simulink model "exp3_5_STATE_SPACE_LQR_FREQ"  (R2020b)
settings: Solver=ode3  StartTime=0.0  StopTime=10  FixedStep=0.001  RelTol=1e-3
undefined symbols (not defined in the file): Aq, Bq, denH_w, DiscIntNeverNeededParam, enable_integral_action, K_ih, K_ss, National_Instruments, Nu, numH_w, Nx, PCI, sens, step_height, step_start_time, Ts
libraries: sldrtlib x3, simulink x3
settings Model: SimulationMode=external  ExtModeTrigDuration=150000  Creator=controlsystemsuser  LastModifiedBy=grandinmat
settings DataIOCC: ReturnWorkspaceOutputs=off
settings RTWCC: Description=Simulink Desktop Real-Time  SystemTargetFile=sldrt.tlc  TemplateMakefile=sldrt.tmf  RTWCompilerOptimization=on
settings CodeAppCC: MaxIdLength=95
settings SimulinkDesktopRealTimeCC: TargetPreCompLibLocation=C:\Program Files\MATLAB\R2020b\toolbox\sldrt\lib\win64

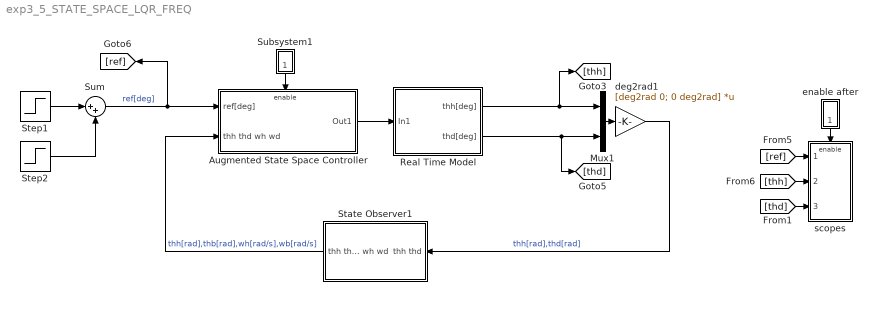
== system exp3_5_STATE_SPACE_LQR_FREQ ==
  Augmented State Space Controller : Subsystem
  Mux1 : Mux  Inputs=2
  Real Time Model : Subsystem
  State Observer1 : Subsystem
  Step1 : Step  Time=step_start_time  After=step_height  SampleTime=0
  Step2 : Step  Time=step_start_time+5  After=-step_height  SampleTime=0
  Subsystem1 : Subsystem
  Sum : Sum  Inputs=|++
  deg2rad1 : Gain  Gain=[deg2rad 0; 0 deg2rad]  Multiplication=Matrix(K*u) (u vector)
  enable after : Subsystem
  scopes : Subsystem
  wires:
  Step2/1 -> Sum/2
  Sum/1 -> Augmented State Space Controller/1(ref[deg]), [ref]  "ref[deg]"
  Step1/1 -> Sum/1
  State Observer1/1(thh thd wh wd) -> Augmented State Space Controller/2(thh thd wh wd)  "thh[rad],thb[rad],wh[rad/s],wb[rad/s]"
  Augmented State Space Controller/1(Out1) -> Real Time Model/1(In1)
  Mux1/1 -> deg2rad1/1
  deg2rad1/1 -> State Observer1/1(thh thd)  "thh[rad],thd[rad]"
  Subsystem1/1(0.8) -> Augmented State Space Controller/Enable
  Real Time Model/2(thd[deg]) -> [thd], Mux1/2
  Real Time Model/1(thh[deg]) -> [thh], Mux1/1
  [thh] -> scopes/2(thh[deg])
  [ref] -> scopes/1(ref[deg])
  [thd] -> scopes/3(thd[deg])
  enable after/1(1.0 s) -> scopes/Enable

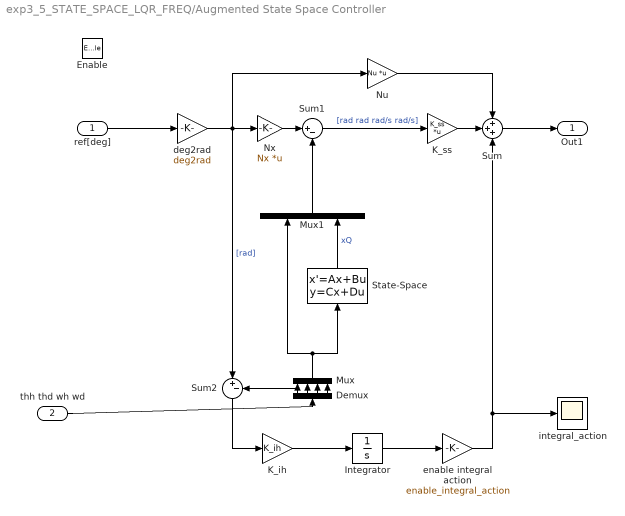
== system exp3_5_STATE_SPACE_LQR_FREQ/Augmented State Space Controller ==
  ref[deg] : Inport
  thh thd wh wd : Inport  Port=2
  Enable : EnablePort
  Demux : Demux
  Integrator : Integrator
  K_ih : Gain  Gain=K_ih
  K_ss : Gain  Gain=K_ss  Multiplication=Matrix(K*u) (u vector)
  Mux : Mux
  Mux1 : Mux  Inputs=2
  Nu : Gain  Gain=Nu  Multiplication=Matrix(K*u) (u vector)
  Nx : Gain  Gain=Nx  Multiplication=Matrix(K*u) (u vector)
  State-Space : StateSpace  A=Aq  B=Bq  C=eye(2,2)  D=zeros(2,4)  InitialCondition=0
  Sum : Sum  Inputs=+++
  Sum1 : Sum  Inputs=|+-
  Sum2 : Sum  Inputs=|+-
  deg2rad : Gain  Gain=deg2rad
  enable integral action : Gain  Gain=enable_integral_action
  integral_action : Scope
  Out1 : Outport
  wires:
  deg2rad/1 -> Nx/1, Nu/1, Sum2/1  "[rad]"
  K_ss/1 -> Sum/2
  Nx/1 -> Sum1/1
  ref[deg]/1 -> deg2rad/1
  Nu/1 -> Sum/1
  Sum/1 -> Out1/1
  Sum1/1 -> K_ss/1  "[rad rad rad/s rad/s]"
  Demux/1 -> Mux/1, Sum2/2
  Demux/2 -> Mux/2
  Demux/3 -> Mux/3
  Demux/4 -> Mux/4
  thh thd wh wd/1 -> Demux/1
  Sum2/1 -> K_ih/1
  enable integral action/1 -> Sum/3, integral_action/1
  Mux/1 -> State-Space/1, Mux1/1
  State-Space/1 -> Mux1/2  "xQ"
  Mux1/1 -> Sum1/2
  K_ih/1 -> Integrator/1
  Integrator/1 -> enable integral action/1

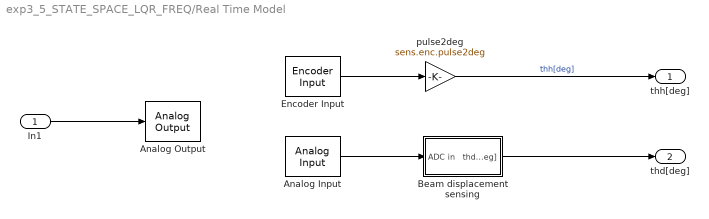
== system exp3_5_STATE_SPACE_LQR_FREQ/Real Time Model ==
  In1 : Inport
  Analog Input : sldrtlib/Analog Input  SampleTime=0.001  MaxMissedTicks=10  ShowMissedTicks=off  YieldWhenWaiting=off  DrvName=National_Instruments/PCI-6221  DrvAddress=4294967295  DrvOptions=[0 0 0 2 0]  Channels=[3,4]  RangeMode=1  VoltRange=2  DataType=1
      settings: AttributesFormatString=National Instruments\nPCI-6221 [auto]
  Analog Output : sldrtlib/Analog Output  SampleTime=0.001  MaxMissedTicks=10  ShowMissedTicks=off  YieldWhenWaiting=off  DrvName=National_Instruments/PCI-6221  DrvAddress=4294967295  DrvOptions=[0 0 0 2 0]  Channels=1  RangeMode=1  VoltRange=1  InitialValue=0  FinalValue=0
      settings: AttributesFormatString=National Instruments\nPCI-6221 [auto]
  Beam displacement sensing : Subsystem
  Encoder Input : sldrtlib/Encoder Input  SampleTime=0.001  MaxMissedTicks=10  ShowMissedTicks=off  YieldWhenWaiting=off  DrvName=National_Instruments/PCI-6221  DrvAddress=4294967295  DrvOptions=[0 0 0 2 0]  Channels=1  QuadMode=3  IndexPulse=1  InputFilter=Inf  DataType=1
      settings: AttributesFormatString=National Instruments\nPCI-6221 [auto]
  pulse2deg : Gain  Gain=sens.enc.pulse2deg
  thh[deg] : Outport
  thd[deg] : Outport  Port=2
  wires:
  Encoder Input/1 -> pulse2deg/1
  Beam displacement sensing/1(thd[deg]) -> thd[deg]/1
  Analog Input/1 -> Beam displacement sensing/1(ADC in)
  pulse2deg/1 -> thh[deg]/1  "thh[deg]"
  In1/1 -> Analog Output/1

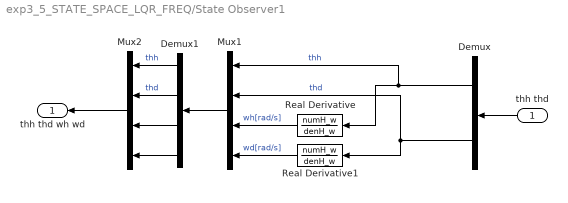
== system exp3_5_STATE_SPACE_LQR_FREQ/State Observer1 ==
  thh thd : Inport
  Demux : Demux  Outputs=2
  Demux1 : Demux
  Mux1 : Mux
  Mux2 : Mux
  Real Derivative : TransferFcn  Numerator=numH_w  Denominator=denH_w
  Real Derivative1 : TransferFcn  Numerator=numH_w  Denominator=denH_w
  thh thd wh wd : Outport
  wires:
  Real Derivative/1 -> Mux1/3  "wh[rad/s]"
  Demux/1 -> Real Derivative/1, Mux1/1  "thh"
  thh thd/1 -> Demux/1
  Real Derivative1/1 -> Mux1/4  "wd[rad/s]"
  Demux/2 -> Mux1/2, Real Derivative1/1  "thd"
  Mux2/1 -> thh thd wh wd/1
  Mux1/1 -> Demux1/1
  Demux1/1 -> Mux2/1  "thh"
  Demux1/2 -> Mux2/2  "thd"
  Demux1/3 -> Mux2/3
  Demux1/4 -> Mux2/4

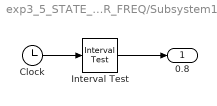
== system exp3_5_STATE_SPACE_LQR_FREQ/Subsystem1 ==
  Clock : Clock
  Interval Test : simulink/Logic and Bit Operations/Interval Test  IntervalClosedRight=on  uplimit=inf  IntervalClosedLeft=on  lowlimit=0.8  OutDataTypeStr=boolean
  0.8 : Outport
  wires:
  Clock/1 -> Interval Test/1
  Interval Test/1 -> 0.8/1

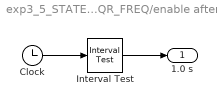
== system exp3_5_STATE_SPACE_LQR_FREQ/enable after ==
  Clock : Clock
  Interval Test : simulink/Logic and Bit Operations/Interval Test  IntervalClosedRight=on  uplimit=inf  IntervalClosedLeft=on  lowlimit=1  OutDataTypeStr=boolean
  1.0 s : Outport
  wires:
  Interval Test/1 -> 1.0 s/1
  Clock/1 -> Interval Test/1

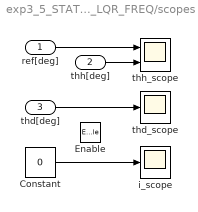
== system exp3_5_STATE_SPACE_LQR_FREQ/scopes ==
  ref[deg] : Inport
  thh[deg] : Inport  Port=2
  thd[deg] : Inport  Port=3
  Enable : EnablePort
  Constant : Constant  Value=0
  i_scope : Scope
  thd_scope : Scope
  thh_scope : Scope  NumInputPorts=2
  wires:
  thd[deg]/1 -> thd_scope/1
  Constant/1 -> i_scope/1
  thh[deg]/1 -> thh_scope/2
  ref[deg]/1 -> thh_scope/1

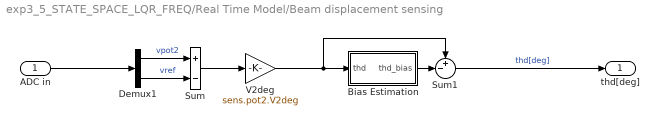
== system exp3_5_STATE_SPACE_LQR_FREQ/Real Time Model/Beam displacement sensing ==
  ADC in : Inport
  Bias Estimation : Subsystem
  Demux1 : Demux  Outputs=2
  Sum : Sum  Inputs=+-
  Sum1 : Sum  Inputs=+-|
  V2deg : Gain  Gain=sens.pot2.V2deg
  thd[deg] : Outport
  wires:
  Bias Estimation/1(thd_bias) -> Sum1/2
  Sum/1 -> V2deg/1
  Demux1/1 -> Sum/1  "vpot2"
  Demux1/2 -> Sum/2  "vref"
  Sum1/1 -> thd[deg]/1  "thd[deg]"
  V2deg/1 -> Sum1/1, Bias Estimation/1(thd)
  ADC in/1 -> Demux1/1

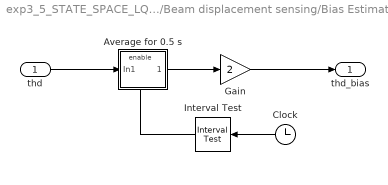
== system exp3_5_STATE_SPACE_LQR_FREQ/Real Time Model/Beam displacement sensing/Bias Estimation ==
  thd : Inport
  Average for 0.5 s : Subsystem
  Clock : Clock
  Gain : Gain  Gain=2
  Interval Test : simulink/Logic and Bit Operations/Interval Test  IntervalClosedRight=on  uplimit=0.7  IntervalClosedLeft=on  lowlimit=0.2  OutDataTypeStr=boolean
  thd_bias : Outport
  wires:
  Interval Test/1 -> Average for 0.5 s/Enable
  thd/1 -> Average for 0.5 s/1(In1)
  Clock/1 -> Interval Test/1
  Average for 0.5 s/1(Out1) -> Gain/1
  Gain/1 -> thd_bias/1

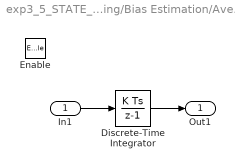
== system exp3_5_STATE_SPACE_LQR_FREQ/Real Time Model/Beam displacement sensing/Bias Estimation/Average for 0.5 s ==
  In1 : Inport
  Enable : EnablePort
  Discrete-Time Integrator : DiscreteIntegrator  SampleTime=Ts  ICPrevOutput=DiscIntNeverNeededParam  ICPrevScaledInput=DiscIntNeverNeededParam
  Out1 : Outport
  wires:
  In1/1 -> Discrete-Time Integrator/1
  Discrete-Time Integrator/1 -> Out1/1
